simulink model "KinematicBicycleModelAttempt"  (R2023b)
settings: Solver=VariableStepAuto  StartTime=0.0  StopTime=50  RelTol=1e-3
libraries: simulink x2, slpidlib x1
settings Model: Creator=binyh  LastModifiedBy=binyh

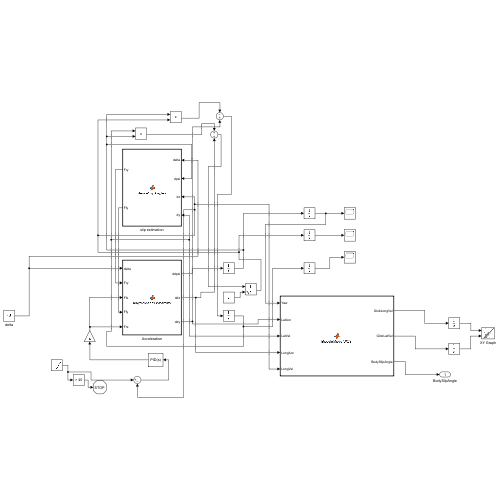
[thumbnail: Simulink's stored preview of the top-level diagram]
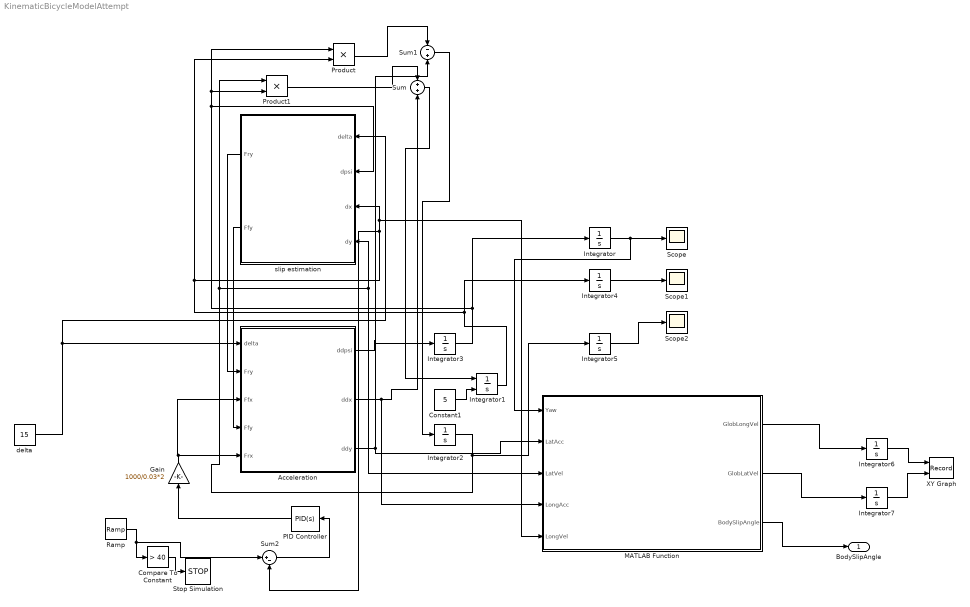
== system KinematicBicycleModelAttempt ==
  Acceleration : MATLAB Function  TreatAsAtomicUnit=on
  Compare To Constant : simulink/Logic and Bit Operations/Compare To Constant  relop=>  const=40  OutDataTypeStr=boolean
  Constant1 : Constant  Value=5
  Gain : Gain  Gain=1000/0.03*2
  Integrator{,2..7} (7 alike) : Integrator
  Integrator1 : Integrator  InitialConditionSource=external
  MATLAB Function : MATLAB Function  TreatAsAtomicUnit=on
  PID Controller : slpidlib/PID Controller  Controller=PID  Form=Parallel  TimeDomain=Continuous-time  UseExternalTs=off  SampleTime=-1  IntegratorMethod=Forward Euler  FilterMethod=Forward Euler  ControllerParametersSource=internal  P=-5.3625761532715e-05  I=-3.1284887958269e-07  UseKiTs=off  D=-0.00204236477981526  N=114.28279760416  UseFilter=on  TunerSelectOption=Transfer Function Based (PID Tuner App)  InitialConditionSource=internal  InitialConditionForIntegrator=0  InitialConditionForFilter=0  DifferentiatorICPrevScaledInput=0  ExternalReset=none  TrackingMode=off  Kt=1  LimitOutput=off  SatLimitsSource=internal  UpperSaturationLimit=inf  LowerSaturationLimit=-inf  LinearizeAsGain=on  AntiWindupMode=none  Kb=1  LimitIntegrator=off  UpperIntegratorSaturationLimit=inf  LowerIntegratorSaturationLimit=-inf  POutMin=[]  POutMax=[]  IOutMin=[]  IOutMax=[]  DOutMin=[]  DOutMax=[]  NOutMin=[]  NOutMax=[]  SumOutMin=[]  SumOutMax=[]  SaturationOutMin=[]  SaturationOutMax=[]  PParamMin=[]  PParamMax=[]  IParamMin=[]  IParamMax=[]  DParamMin=[]  DParamMax=[]  NParamMin=[]  NParamMax=[]  KbParamMin=[]  KbParamMax=[]  KtParamMin=[]  KtParamMax=[]  KbOutMin=[]  KbOutMax=[]  KtOutMin=[]  KtOutMax=[]  IntegratorOutMin=[]  IntegratorOutMax=[]  FilterOutMin=[]  FilterOutMax=[]  SumI1OutMin=[]  SumI1OutMax=[]  SumI2OutMin=[]  SumI2OutMax=[]  SumI3OutMin=[]  SumI3OutMax=[]  SumI4OutMin=[]  SumI4OutMax=[]  SumDOutMin=[]  SumDOutMax=[]  DifferentiatorOutMin=[]  DifferentiatorOutMax=[]  FilterDiffOutCoefMin=[]  FilterDiffOutCoefMax=[]  ReciprocalOutMin=[]  ReciprocalOutMax=[]  SumDenOutMin=[]  SumDenOutMax=[]  SumNumOutMin=[]  SumNumOutMax=[]  DivideOutMin=[]  DivideOutMax=[]  UdiffTsProdOutMin=[]  UdiffTsProdOutMax=[]  NTsProdOutMin=[]  NTsProdOutMax=[]  UintegralTsProdOutMin=[]  UintegralTsProdOutMax=[]  UngainTsProdOutMin=[]  UngainTsProdOutMax=[]  ClampingZeroOutDataTypeStr=Inherit: Inherit via back propagation  ClampingZeroOutMin=[]  ClampingZeroOutMax=[]  FilterDenConstantOutDataTypeStr=Inherit: Inherit via back propagation  FilterDenConstantOutMin=[]  FilterDenConstantOutMax=[]  PCopyOutDataTypeStr=Inherit: Inherit via back propagation  PCopyOutMin=[]  PCopyOutMax=[]  NCopyOutDataTypeStr=Inherit: Inherit via back propagation  NCopyOutMin=[]  NCopyOutMax=[]  IntegratorContinuousStateAttributes=''  IntegratorStateMustResolveToSignalObject=off  IntegratorRTWStateStorageClass=Auto  FilterContinuousStateAttributes=''  FilterStateMustResolveToSignalObject=off  FilterRTWStateStorageClass=Auto  ParallelPVariant=InternalParameters  IdealPVariant=Disabled  IVariant=InternalParameters  DVariant=InternalParameters  IntegratorVariant=Continuous  SatVariant=Disabled  AWVariant=Passthrough  PCopyVariant=Disabled  TRVariant=Disabled  FdbkBlocksVariant=Forward  IdealPFdbkVariant=Disabled  SatFdbkVariant=Disabled  DerivativeFilterVariant=ContFilter  NVariant=InternalParameters  NCopyVariant=Disabled  FilterICVariant=InternalICsFilter  IntegratorICVariant=InternalICs  ExternalResetVariant=Disabled  TRSumVariant=Passthrough  SumFdbkVariant=Disabled  SumVariant=Sum_PID  TsampFilterVariant=InternalTs  TsampNgainVariant=Passthrough  TsampIntegralVariant=Disabled_SignalSpec  ExternalSaturationOutDataTypeStr=Inherit: Same as second input
  Product : Product
  Product1 : Product
  Ramp : simulink/Sources/Ramp  slope=0.05  start=0  InitialOutput=5
  Scope : Scope
  Scope1 : Scope
  Scope2 : Scope
  Stop Simulation : Stop
  Sum : Sum
  Sum1 : Sum  Inputs=-+
  Sum2 : Sum  Inputs=|+-
  XY Graph : Record  FileSettingsInternal="{\"entries\":[{\"content\":{\"excelSettings\":{\"content\":{},\"type\":\"Streamout.ExcelSettings\"}},\"type\":\"Streamout.FileSettingStorage\",\"uuid\":\"\"}],\"packageUris\":[\"http:\\/\\/schema.mathworks.com\\/mf0\\/streamout_blocks\\/R2020a\"],\"version\":\"1.0\"}"  Layout=[1 1]  SignalsInternal="{\"entries\":[{\"content\":{\"signals\":[{\"content\":{\"blockPath\":[],\"dimensions\":[1],\"domain\":\"\",\"lineColor\":\"#a2142f\",\"plots\":[1],\"port\":1,\"sid\":[\"\"],\"signalID\":5651,\"signalName\":\"Integrator6\"},\"type\":\"RecordBlkView.Signal\",\"uuid\":\"\"},{\"content\":{\"blockPath\":[],\"dimensions\":[1],\"domain\":\"\",\"lineColor\":\"#139fff\",\"plots\":[1],\"port\":2,\"sid\":[\"\"],\"signalID\":5655,\"signalName\":\"Integrator7\"},\"type\":\"RecordBlkView.Signal\",\"uuid\":\"\"}]},\"type\":\"RecordBlkView.InputSignals\",\"uuid\":\"\"}],\"packageUris\":[\"http:\\/\\/schema.mathworks.com\\/mf0\\/streamout_blocks\\/R2020a\"],\"version\":\"1.0\"}"  VisualizationBindings="{\"xyplotplugin\":{\"info\":[{\"series\":[{\"bindingParametersList\":[{\"parameter\":\"X-Axis\",\"signalID\":5651,\"signalName\":\"Integrator6\"},{\"parameter\":\"Y-Axis\",\"signalID\":5655,\"signalName\":\"Integrator7\"}],\"seriesID\":56440}],\"subplotID\":1}]}}"  CompatibilityTag=XY
  delta : Constant  Value=15
  slip estimation : MATLAB Function  TreatAsAtomicUnit=on
  BodySlipAngle : Outport
  wires:
  delta/1 -> slip estimation/1(delta), Acceleration/1(delta)
  Acceleration/1(ddpsi) -> Integrator3/1
  Acceleration/2(ddx) -> MATLAB Function/4(LongAcc), Sum/2
  Integrator3/1 -> Integrator/1, Product/1, Product1/2, slip estimation/2(dpsi)
  Integrator1/1 -> Integrator4/1, Product/2, Sum2/2, slip estimation/3(dx), MATLAB Function/5(LongVel)
  Integrator2/1 -> Integrator5/1, Product1/1, slip estimation/4(dy), MATLAB Function/3(LatVel)
  slip estimation/2(Ffy) -> Acceleration/4(Ffy)
  slip estimation/1(Fry) -> Acceleration/2(Fry)
  Integrator/1 -> MATLAB Function/1(Yaw), Scope/1
  Integrator4/1 -> Scope1/1
  Integrator5/1 -> Scope2/1
  Product1/1 -> Sum/1
  Sum/1 -> Integrator1/1
  Acceleration/3(ddy) -> Sum1/2, MATLAB Function/2(LatAcc)
  Product/1 -> Sum1/1
  Sum1/1 -> Integrator2/1
  Ramp/1 -> Sum2/1, Compare To Constant/1
  Sum2/1 -> PID Controller/1
  MATLAB Function/3(BodySlipAngle) -> BodySlipAngle/1
  MATLAB Function/1(GlobLongVel) -> Integrator6/1
  MATLAB Function/2(GlobLatVel) -> Integrator7/1
  Integrator6/1 -> XY Graph/1
  Integrator7/1 -> XY Graph/2
  Constant1/1 -> Integrator1/2
  Compare To Constant/1 -> Stop Simulation/1
  PID Controller/1 -> Gain/1
  Gain/1 -> Acceleration/3(Ffx), Acceleration/5(Frx)

== matlab function KinematicBicycleModelAttempt/slip estimation ==
  data: delta input; Fry output; dpsi input; dx input; Ffy output; dy input
function [Fry, Ffy] = deriveSlipAngles(delta, dpsi, dx, dy)    
    % Calculating the lateral forces on the front and rear wheels of model 
    % based on the slip angles derived from the vehicle's kinematics. 
    % Takes into account the steering angle (delta), yaw
    % rate, and long and lat velocities.

    % Parameters:
    L = 1.525;          % Total wheelbase: distance from CG to front wheel.
    PercentFront = 0.6; % Percentage distribution of wheelbase at the front.
    k = 400;            % Tire stiffness coefficient.

    % Calculate distances from CG to front and rear wheels.
    Lf = L * (1 - PercentFront); % Distance to the front wheel.
    Lr = L * PercentFront;       % Distance to the rear wheel.

    % Slip angle calculation:
    % angle between the direction of the wheel and direction of travel. 
    % Calculating the front slip angle (alphaF).
    % determined by the steering angle and the difference between the 
    % lateral and longitudinal velocities at the front wheel.
    alphaF = delta - atan2d(dy - (Lf * dpsi), dx);

    % Calculating the rear slip angle (alphaR).
    % Similar to the front, but only influenced by the velocities at the rear wheel.
    alphaR = -atan2d(dy - (Lr * dpsi), dx);
    % Note: The negative sign accounts for the coordinate system used.

    % Calculating the lateral forces based on the slip angles.
    % Tire lateral forces are proportional to the slip angles, with the proportionality
    % constant being the tire stiffness 'k'.
    Fry = k * alphaR; % Lateral force at the rear wheel.
    Ffy = k * alphaF; % Lateral force at the front wheel.
end

== matlab function KinematicBicycleModelAttempt/Acceleration ==
  data: ddpsi output; delta input; ddx output; ddy output; Fry input; Ffx input; Ffy input; Frx input
function [ddpsi, ddx, ddy] = bicycleModelDynamics(delta, Fry, Ffx, Ffy, Frx)
    % Calculating the second derivatives of yaw angle, long. displacement,
    % lat. displacement based on forces and steering angle.

    % Parameters (arbitrary values)
    L = 1.525; % Total wheelbase: distance from center of gravity (CG) to front wheel.
    I = 2.75;   % Vehicle's moment of inertia.
    m = 275;   % Mass of the vehicle in kg.
    PercentFront = 0.6; % Percentage distribution of wheelbase at the front.

    % Dynamics equations
    % Calculating the effective distances to the front (Lf) and rear (Lr) wheels from CG.
    Lf = L * (1 - PercentFront); % Distance from CG to front wheel.
    Lr = L * PercentFront;       % Distance from CG to rear wheel.

    % Calculating the second derivative of yaw angle (ddpsi).
    % It's a measure of how quickly the vehicle is rotating about its vertical axis.
    ddpsi = (Lr * Fry - Lf * (Ffx * sind(delta) + Ffy * sind(delta))) / I;

    % Calculating the second derivative of longitudinal displacement (ddx).
    % This is the acceleration in the vehicle's forward direction.
    ddx = (Frx + Ffx * cosd(delta) - Ffy * sind(delta)) / m;

    % Calculating the second derivative of lateral displacement (ddy).
    % This is the acceleration perpendicular to the vehicle's forward direction.
    ddy = (Fry + Ffx * sind(delta) + Ffy * sind(delta)) / m;
    
end

== matlab function KinematicBicycleModelAttempt/MATLAB Function ==
  data: Yaw input; GlobLongVel output; LatAcc input; LatVel input; LongAcc input; LongVel input; GlobLatVel output; BodySlipAngle output
function [GlobLongVel, GlobLatVel, BodySlipAngle] = ...
    BicycleModelWCS( Yaw, LatAcc, LatVel, LongAcc, LongVel )

%% WCS - World Coordinate System Calculations
% 
% Inputs:
%  Yaw     - (n,1 numeric) Yaw                       {psi} [rad]
%  LatAcc  - (n,1 numeric) Lateral Acceleration      {y_ddot} [m/s^2]
%  LatVel  - (n,1 numeric) Lateral Velocity          {y_dot} [m/s]
%  LongAcc - (n,1 numeric) Longitudinal Acceleration {x_ddot} [m/s^2]
%  LongVel - (n,1 numeric) Longitudinal Velocity     {x_dot} [m/s]
% 
% Outputs:
%  GlobLongVel   - (n,1 numeric) Global Longitudial Velocity {X_dot} [m/s]
%  GlobLatVel    - (n,1 numeric) Golbal Lateral Velocity     {Y_dot} [m/s]
%  BodySlipAngle - (n,1 numeric) Body Slip Angle             {beta} [degrees]
%  
% Notes:
% Naming convention for R still not in place
%
% Author(s): 
% Tristan Pham (atlpham@ucdavis.edu) [Sep 2020 - Jun 2021] 

% Last Updated: 27-Mar-2021


    
%% Computation

% Global Velocity
GlobLongVel = LongVel .* cosd( Yaw ) - LatVel .* sind( Yaw );
GlobLatVel = LongVel .* sind( Yaw ) + LatVel .* cosd( Yaw );  
                 

% Body Slip
BodySlipAngle = atan2d( LatVel, LongVel );

end
